simulink model "draft2"  (R2020b)
settings: Solver=VariableStepAuto  StartTime=0.0  StopTime=10.0  FixedStep=0.0001  MaxStep=0.2  RelTol=1e-3  AbsTol=1e-3  EnableMultiTasking=on
model workspace (MAT data in the model file):
  c = 0.1
  k : Simulink.Parameter (value not decoded)
libraries: nesl_utility x118, sm_lib x40, simulink x5, simulink_extras x5, fl_lib x1
(part 5 of 5)

== system draft2/T8/LB torque feedback L4 ==
  Gain4 : Gain  Gain=-1
  PS-Simulink Converter8 : nesl_utility/PS-Simulink Converter  PhysicalDomain=network_engine_domain  SubClassName=ps_output  LeftPortType=input  RightPortType=output  PseudoPeriodic=off  Frequencies=[]  Unit=inherit  AffineConversion=off
  Simulink-PS Converter5 : nesl_utility/Simulink-PS Converter  PhysicalDomain=network_engine_domain  SubClassName=ps_input  LeftPortType=input  RightPortType=output  PseudoPeriodic=off  Frequencies=[]  NoiseDistribution=none  NoiseParameters=[]  Unit=1  AffineConversion=off  FilteringAndDerivatives=provide  SimscapeFilterOrder=1  InputFilterTimeConstant=0.001  UdotUserProvided=0
  peacewise torque profile4 : MATLAB Function  TreatAsAtomicUnit=on
  LB rot : PMIOPort  Side=Left
  LB torque : PMIOPort  Port=2  Side=Right
  wires:
  peacewise torque profile4/1(torque) -> Gain4/1
  PS-Simulink Converter8/1 -> peacewise torque profile4/1(u)
  Gain4/1 -> Simulink-PS Converter5/1
  connections:
  LB rot/RConn1 -- PS-Simulink Converter8/LConn1
  Simulink-PS Converter5/RConn1 -- LB torque/RConn1

== system draft2/T9/AR torque feedback L4 ==
  Gain5 : Gain  Gain=-1
  PS-Simulink Converter9 : nesl_utility/PS-Simulink Converter  PhysicalDomain=network_engine_domain  SubClassName=ps_output  LeftPortType=input  RightPortType=output  PseudoPeriodic=off  Frequencies=[]  Unit=inherit  AffineConversion=off
  Simulink-PS Converter6 : nesl_utility/Simulink-PS Converter  PhysicalDomain=network_engine_domain  SubClassName=ps_input  LeftPortType=input  RightPortType=output  PseudoPeriodic=off  Frequencies=[]  NoiseDistribution=none  NoiseParameters=[]  Unit=1  AffineConversion=off  FilteringAndDerivatives=provide  SimscapeFilterOrder=1  InputFilterTimeConstant=0.001  UdotUserProvided=0
  peacewise torque profile5 : MATLAB Function  TreatAsAtomicUnit=on
  AR rot : PMIOPort  Side=Left
  AR torque : PMIOPort  Port=2  Side=Right
  wires:
  PS-Simulink Converter9/1 -> peacewise torque profile5/1(u)
  peacewise torque profile5/1(torque) -> Gain5/1
  Gain5/1 -> Simulink-PS Converter6/1
  connections:
  PS-Simulink Converter9/LConn1 -- AR rot/RConn1
  AR torque/RConn1 -- Simulink-PS Converter6/RConn1

== system draft2/T9/FE torque feedback L4 ==
  Gain7 : Gain  Gain=-1
  PS-Simulink Converter5 : nesl_utility/PS-Simulink Converter  PhysicalDomain=network_engine_domain  SubClassName=ps_output  LeftPortType=input  RightPortType=output  PseudoPeriodic=off  Frequencies=[]  Unit=inherit  AffineConversion=off
  Simulink-PS Converter4 : nesl_utility/Simulink-PS Converter  PhysicalDomain=network_engine_domain  SubClassName=ps_input  LeftPortType=input  RightPortType=output  PseudoPeriodic=off  Frequencies=[]  NoiseDistribution=none  NoiseParameters=[]  Unit=1  AffineConversion=off  FilteringAndDerivatives=provide  SimscapeFilterOrder=1  InputFilterTimeConstant=0.001  UdotUserProvided=0
  peacewise torque profile1 : MATLAB Function  TreatAsAtomicUnit=on
  FE rot : PMIOPort  Side=Left
  FE torque : PMIOPort  Port=2  Side=Right
  wires:
  PS-Simulink Converter5/1 -> peacewise torque profile1/1(u)
  peacewise torque profile1/1(torque) -> Gain7/1
  Gain7/1 -> Simulink-PS Converter4/1
  connections:
  FE rot/RConn1 -- PS-Simulink Converter5/LConn1
  FE torque/RConn1 -- Simulink-PS Converter4/RConn1

== system draft2/T9/LB torque feedback L4 ==
  Gain4 : Gain  Gain=-1
  PS-Simulink Converter8 : nesl_utility/PS-Simulink Converter  PhysicalDomain=network_engine_domain  SubClassName=ps_output  LeftPortType=input  RightPortType=output  PseudoPeriodic=off  Frequencies=[]  Unit=inherit  AffineConversion=off
  Simulink-PS Converter5 : nesl_utility/Simulink-PS Converter  PhysicalDomain=network_engine_domain  SubClassName=ps_input  LeftPortType=input  RightPortType=output  PseudoPeriodic=off  Frequencies=[]  NoiseDistribution=none  NoiseParameters=[]  Unit=1  AffineConversion=off  FilteringAndDerivatives=provide  SimscapeFilterOrder=1  InputFilterTimeConstant=0.001  UdotUserProvided=0
  peacewise torque profile4 : MATLAB Function  TreatAsAtomicUnit=on
  LB rot : PMIOPort  Side=Left
  LB torque : PMIOPort  Port=2  Side=Right
  wires:
  Gain4/1 -> Simulink-PS Converter5/1
  PS-Simulink Converter8/1 -> peacewise torque profile4/1(u)
  peacewise torque profile4/1(torque) -> Gain4/1
  connections:
  Simulink-PS Converter5/RConn1 -- LB torque/RConn1
  LB rot/RConn1 -- PS-Simulink Converter8/LConn1

== matlab function draft2/L1/LB torque feedback L4/peacewise torque profile4 ==
  data: u input; torque output
function torque = T(u)
torque = 0;
if (u >= 15)
    torque= -0.0015*1*(57.295*15)^4 + 0.1326*(57.295*15)^3 -0.3477*(57.295*15)^2 + 0.499*(57.295*15);
 
elseif (u >= -15 && u<= 15)
    torque= -0.0015*(57.295*u)^4 + 0.1326*(57.295*u)^3 -0.3477*(57.295*u)^2 + 0.499*(57.295*u)   ;
    
elseif (u <= -15)
   torque= -0.0015*1*(57.295*-15)^4 + 0.1326*(57.295*-15)^3 -0.3477*(57.295*-15)^2 + 0.499*(57.295*-15);
end

== matlab function draft2/T12/AR torque feedback L4/peacewise torque profile5 ==
  data: u input; torque output
function torque = T(u)
torque = 0;
if (u >= 15)
    torque= -0.0015*1*(57.295*15)^4 + 0.1326*(57.295*15)^3 -0.3477*(57.295*15)^2 + 0.499*(57.295*15);
 
elseif (u >= -15 && u<= 15)
    torque= -0.0015*(57.295*u)^4 + 0.1326*(57.295*u)^3 -0.3477*(57.295*u)^2 + 0.499*(57.295*u)   ;
    
elseif (u <= -15)
   torque= -0.0015*1*(57.295*-15)^4 + 0.1326*(57.295*-15)^3 -0.3477*(57.295*-15)^2 + 0.499*(57.295*-15);
end

== matlab function draft2/T12/FE torque feedback L4/peacewise torque profile1 ==
  data: u input; torque output
function torque = T(u)
torque = 0;
if (u >= 15)
    torque= -0.0015*1*(57.295*15)^4 + 0.1326*(57.295*15)^3 -0.3477*(57.295*15)^2 + 0.499*(57.295*15);
 
elseif (u >= -15 && u<= 15)
    torque= -0.0015*(57.295*u)^4 + 0.1326*(57.295*u)^3 -0.3477*(57.295*u)^2 + 0.499*(57.295*u)   ;
    
elseif (u <= -15)
   torque= -0.0015*1*(57.295*-15)^4 + 0.1326*(57.295*-15)^3 -0.3477*(57.295*-15)^2 + 0.499*(57.295*-15);
end

== matlab function draft2/T12/LB torque feedback L4/peacewise torque profile4 ==
  data: u input; torque output
function torque = T(u)
torque = 0;
if (u >= 15)
    torque= -0.0015*1*(57.295*15)^4 + 0.1326*(57.295*15)^3 -0.3477*(57.295*15)^2 + 0.499*(57.295*15);
 
elseif (u >= -15 && u<= 15)
    torque= -0.0015*(57.295*u)^4 + 0.1326*(57.295*u)^3 -0.3477*(57.295*u)^2 + 0.499*(57.295*u)   ;
    
elseif (u <= -15)
   torque= -0.0015*1*(57.295*-15)^4 + 0.1326*(57.295*-15)^3 -0.3477*(57.295*-15)^2 + 0.499*(57.295*-15);
end

== matlab function draft2/T11/AR torque feedback L4/peacewise torque profile5 ==
  data: u input; torque output
function torque = T(u)
torque = 0;
if (u >= 15)
    torque= -0.0015*1*(57.295*15)^4 + 0.1326*(57.295*15)^3 -0.3477*(57.295*15)^2 + 0.499*(57.295*15);
 
elseif (u >= -15 && u<= 15)
    torque= -0.0015*(57.295*u)^4 + 0.1326*(57.295*u)^3 -0.3477*(57.295*u)^2 + 0.499*(57.295*u)   ;
    
elseif (u <= -15)
   torque= -0.0015*1*(57.295*-15)^4 + 0.1326*(57.295*-15)^3 -0.3477*(57.295*-15)^2 + 0.499*(57.295*-15);
end

== matlab function draft2/L5/FE torque feedback L5/peacewise torque profile (+- 15 deg) ==
  data: u input; torque output
function torque = T(u)
torque = 0;
if (u >= 15)
    torque= -0.0015*1*(57.295*15)^4 + 0.1326*(57.295*15)^3 -0.3477*(57.295*15)^2 + 0.499*(57.295*15);
 
elseif (u >= -15 && u<= 15)
    torque= -0.0015*(57.295*u)^4 + 0.1326*(57.295*u)^3 -0.3477*(57.295*u)^2 + 0.499*(57.295*u)   ;
    
elseif (u <= -15)
   torque= -0.0015*1*(57.295*-15)^4 + 0.1326*(57.295*-15)^3 -0.3477*(57.295*-15)^2 + 0.499*(57.295*-15);
end

== matlab function draft2/T11/FE torque feedback L4/peacewise torque profile1 ==
  data: u input; torque output
function torque = T(u)
torque = 0;
if (u >= 15)
    torque= -0.0015*1*(57.295*15)^4 + 0.1326*(57.295*15)^3 -0.3477*(57.295*15)^2 + 0.499*(57.295*15);
 
elseif (u >= -15 && u<= 15)
    torque= -0.0015*(57.295*u)^4 + 0.1326*(57.295*u)^3 -0.3477*(57.295*u)^2 + 0.499*(57.295*u)   ;
    
elseif (u <= -15)
   torque= -0.0015*1*(57.295*-15)^4 + 0.1326*(57.295*-15)^3 -0.3477*(57.295*-15)^2 + 0.499*(57.295*-15);
end

== matlab function draft2/T11/LB torque feedback L4/peacewise torque profile4 ==
  data: u input; torque output
function torque = T(u)
torque = 0;
if (u >= 15)
    torque= -0.0015*1*(57.295*15)^4 + 0.1326*(57.295*15)^3 -0.3477*(57.295*15)^2 + 0.499*(57.295*15);
 
elseif (u >= -15 && u<= 15)
    torque= -0.0015*(57.295*u)^4 + 0.1326*(57.295*u)^3 -0.3477*(57.295*u)^2 + 0.499*(57.295*u)   ;
    
elseif (u <= -15)
   torque= -0.0015*1*(57.295*-15)^4 + 0.1326*(57.295*-15)^3 -0.3477*(57.295*-15)^2 + 0.499*(57.295*-15);
end

== matlab function draft2/T10/AR torque feedback L4/peacewise torque profile5 ==
  data: u input; torque output
function torque = T(u)
torque = 0;
if (u >= 15)
    torque= -0.0015*1*(57.295*15)^4 + 0.1326*(57.295*15)^3 -0.3477*(57.295*15)^2 + 0.499*(57.295*15);
 
elseif (u >= -15 && u<= 15)
    torque= -0.0015*(57.295*u)^4 + 0.1326*(57.295*u)^3 -0.3477*(57.295*u)^2 + 0.499*(57.295*u)   ;
    
elseif (u <= -15)
   torque= -0.0015*1*(57.295*-15)^4 + 0.1326*(57.295*-15)^3 -0.3477*(57.295*-15)^2 + 0.499*(57.295*-15);
end

== matlab function draft2/T10/FE torque feedback L4/peacewise torque profile1 ==
  data: u input; torque output
function torque = T(u)
torque = 0;
if (u >= 15)
    torque= -0.0015*1*(57.295*15)^4 + 0.1326*(57.295*15)^3 -0.3477*(57.295*15)^2 + 0.499*(57.295*15);
 
elseif (u >= -15 && u<= 15)
    torque= -0.0015*(57.295*u)^4 + 0.1326*(57.295*u)^3 -0.3477*(57.295*u)^2 + 0.499*(57.295*u)   ;
    
elseif (u <= -15)
   torque= -0.0015*1*(57.295*-15)^4 + 0.1326*(57.295*-15)^3 -0.3477*(57.295*-15)^2 + 0.499*(57.295*-15);
end

== matlab function draft2/T10/LB torque feedback L4/peacewise torque profile4 ==
  data: u input; torque output
function torque = T(u)
torque = 0;
if (u >= 15)
    torque= -0.0015*1*(57.295*15)^4 + 0.1326*(57.295*15)^3 -0.3477*(57.295*15)^2 + 0.499*(57.295*15);
 
elseif (u >= -15 && u<= 15)
    torque= -0.0015*(57.295*u)^4 + 0.1326*(57.295*u)^3 -0.3477*(57.295*u)^2 + 0.499*(57.295*u)   ;
    
elseif (u <= -15)
   torque= -0.0015*1*(57.295*-15)^4 + 0.1326*(57.295*-15)^3 -0.3477*(57.295*-15)^2 + 0.499*(57.295*-15);
end

== matlab function draft2/T9/AR torque feedback L4/peacewise torque profile5 ==
  data: u input; torque output
function torque = T(u)
torque = 0;
if (u >= 15)
    torque= -0.0015*1*(57.295*15)^4 + 0.1326*(57.295*15)^3 -0.3477*(57.295*15)^2 + 0.499*(57.295*15);
 
elseif (u >= -15 && u<= 15)
    torque= -0.0015*(57.295*u)^4 + 0.1326*(57.295*u)^3 -0.3477*(57.295*u)^2 + 0.499*(57.295*u)   ;
    
elseif (u <= -15)
   torque= -0.0015*1*(57.295*-15)^4 + 0.1326*(57.295*-15)^3 -0.3477*(57.295*-15)^2 + 0.499*(57.295*-15);
end

== matlab function draft2/T9/FE torque feedback L4/peacewise torque profile1 ==
  data: u input; torque output
function torque = T(u)
torque = 0;
if (u >= 15)
    torque= -0.0015*1*(57.295*15)^4 + 0.1326*(57.295*15)^3 -0.3477*(57.295*15)^2 + 0.499*(57.295*15);
 
elseif (u >= -15 && u<= 15)
    torque= -0.0015*(57.295*u)^4 + 0.1326*(57.295*u)^3 -0.3477*(57.295*u)^2 + 0.499*(57.295*u)   ;
    
elseif (u <= -15)
   torque= -0.0015*1*(57.295*-15)^4 + 0.1326*(57.295*-15)^3 -0.3477*(57.295*-15)^2 + 0.499*(57.295*-15);
end

== matlab function draft2/T9/LB torque feedback L4/peacewise torque profile4 ==
  data: u input; torque output
function torque = T(u)
torque = 0;
if (u >= 15)
    torque= -0.0015*1*(57.295*15)^4 + 0.1326*(57.295*15)^3 -0.3477*(57.295*15)^2 + 0.499*(57.295*15);
 
elseif (u >= -15 && u<= 15)
    torque= -0.0015*(57.295*u)^4 + 0.1326*(57.295*u)^3 -0.3477*(57.295*u)^2 + 0.499*(57.295*u)   ;
    
elseif (u <= -15)
   torque= -0.0015*1*(57.295*-15)^4 + 0.1326*(57.295*-15)^3 -0.3477*(57.295*-15)^2 + 0.499*(57.295*-15);
end

== matlab function draft2/T8/AR torque feedback L4/peacewise torque profile5 ==
  data: u input; torque output
function torque = T(u)
torque = 0;
if (u >= 15)
    torque= -0.0015*1*(57.295*15)^4 + 0.1326*(57.295*15)^3 -0.3477*(57.295*15)^2 + 0.499*(57.295*15);
 
elseif (u >= -15 && u<= 15)
    torque= -0.0015*(57.295*u)^4 + 0.1326*(57.295*u)^3 -0.3477*(57.295*u)^2 + 0.499*(57.295*u)   ;
    
elseif (u <= -15)
   torque= -0.0015*1*(57.295*-15)^4 + 0.1326*(57.295*-15)^3 -0.3477*(57.295*-15)^2 + 0.499*(57.295*-15);
end

== matlab function draft2/T8/FE torque feedback L4/peacewise torque profile1 ==
  data: u input; torque output
function torque = T(u)
torque = 0;
if (u >= 15)
    torque= -0.0015*1*(57.295*15)^4 + 0.1326*(57.295*15)^3 -0.3477*(57.295*15)^2 + 0.499*(57.295*15);
 
elseif (u >= -15 && u<= 15)
    torque= -0.0015*(57.295*u)^4 + 0.1326*(57.295*u)^3 -0.3477*(57.295*u)^2 + 0.499*(57.295*u)   ;
    
elseif (u <= -15)
   torque= -0.0015*1*(57.295*-15)^4 + 0.1326*(57.295*-15)^3 -0.3477*(57.295*-15)^2 + 0.499*(57.295*-15);
end

== matlab function draft2/L5/LB torque feedback L5/peacewise torque profile2 ==
  data: u input; torque output
function torque = T(u)
torque = 0;
if (u >= 15)
    torque= -0.0015*1*(57.295*15)^4 + 0.1326*(57.295*15)^3 -0.3477*(57.295*15)^2 + 0.499*(57.295*15);
 
elseif (u >= -15 && u<= 15)
    torque= -0.0015*(57.295*u)^4 + 0.1326*(57.295*u)^3 -0.3477*(57.295*u)^2 + 0.499*(57.295*u)   ;
    
elseif (u <= -15)
   torque= -0.0015*1*(57.295*-15)^4 + 0.1326*(57.295*-15)^3 -0.3477*(57.295*-15)^2 + 0.499*(57.295*-15);
end

== matlab function draft2/T8/LB torque feedback L4/peacewise torque profile4 ==
  data: u input; torque output
function torque = T(u)
torque = 0;
if (u >= 15)
    torque= -0.0015*1*(57.295*15)^4 + 0.1326*(57.295*15)^3 -0.3477*(57.295*15)^2 + 0.499*(57.295*15);
 
elseif (u >= -15 && u<= 15)
    torque= -0.0015*(57.295*u)^4 + 0.1326*(57.295*u)^3 -0.3477*(57.295*u)^2 + 0.499*(57.295*u)   ;
    
elseif (u <= -15)
   torque= -0.0015*1*(57.295*-15)^4 + 0.1326*(57.295*-15)^3 -0.3477*(57.295*-15)^2 + 0.499*(57.295*-15);
end

== matlab function draft2/T7/AR torque feedback L4/peacewise torque profile5 ==
  data: u input; torque output
function torque = T(u)
torque = 0;
if (u >= 15)
    torque= -0.0015*1*(57.295*15)^4 + 0.1326*(57.295*15)^3 -0.3477*(57.295*15)^2 + 0.499*(57.295*15);
 
elseif (u >= -15 && u<= 15)
    torque= -0.0015*(57.295*u)^4 + 0.1326*(57.295*u)^3 -0.3477*(57.295*u)^2 + 0.499*(57.295*u)   ;
    
elseif (u <= -15)
   torque= -0.0015*1*(57.295*-15)^4 + 0.1326*(57.295*-15)^3 -0.3477*(57.295*-15)^2 + 0.499*(57.295*-15);
end

== matlab function draft2/T7/FE torque feedback L4/peacewise torque profile1 ==
  data: u input; torque output
function torque = T(u)
torque = 0;
if (u >= 15)
    torque= -0.0015*1*(57.295*15)^4 + 0.1326*(57.295*15)^3 -0.3477*(57.295*15)^2 + 0.499*(57.295*15);
 
elseif (u >= -15 && u<= 15)
    torque= -0.0015*(57.295*u)^4 + 0.1326*(57.295*u)^3 -0.3477*(57.295*u)^2 + 0.499*(57.295*u)   ;
    
elseif (u <= -15)
   torque= -0.0015*1*(57.295*-15)^4 + 0.1326*(57.295*-15)^3 -0.3477*(57.295*-15)^2 + 0.499*(57.295*-15);
end

== matlab function draft2/T7/LB torque feedback L4/peacewise torque profile4 ==
  data: u input; torque output
function torque = T(u)
torque = 0;
if (u >= 15)
    torque= -0.0015*1*(57.295*15)^4 + 0.1326*(57.295*15)^3 -0.3477*(57.295*15)^2 + 0.499*(57.295*15);
 
elseif (u >= -15 && u<= 15)
    torque= -0.0015*(57.295*u)^4 + 0.1326*(57.295*u)^3 -0.3477*(57.295*u)^2 + 0.499*(57.295*u)   ;
    
elseif (u <= -15)
   torque= -0.0015*1*(57.295*-15)^4 + 0.1326*(57.295*-15)^3 -0.3477*(57.295*-15)^2 + 0.499*(57.295*-15);
end

== matlab function draft2/T6/AR torque feedback L4/peacewise torque profile5 ==
  data: u input; torque output
function torque = T(u)
torque = 0;
if (u >= 15)
    torque= -0.0015*1*(57.295*15)^4 + 0.1326*(57.295*15)^3 -0.3477*(57.295*15)^2 + 0.499*(57.295*15);
 
elseif (u >= -15 && u<= 15)
    torque= -0.0015*(57.295*u)^4 + 0.1326*(57.295*u)^3 -0.3477*(57.295*u)^2 + 0.499*(57.295*u)   ;
    
elseif (u <= -15)
   torque= -0.0015*1*(57.295*-15)^4 + 0.1326*(57.295*-15)^3 -0.3477*(57.295*-15)^2 + 0.499*(57.295*-15);
end

== matlab function draft2/T6/FE torque feedback L4/peacewise torque profile1 ==
  data: u input; torque output
function torque = T(u)
torque = 0;
if (u >= 15)
    torque= -0.0015*1*(57.295*15)^4 + 0.1326*(57.295*15)^3 -0.3477*(57.295*15)^2 + 0.499*(57.295*15);
 
elseif (u >= -15 && u<= 15)
    torque= -0.0015*(57.295*u)^4 + 0.1326*(57.295*u)^3 -0.3477*(57.295*u)^2 + 0.499*(57.295*u)   ;
    
elseif (u <= -15)
   torque= -0.0015*1*(57.295*-15)^4 + 0.1326*(57.295*-15)^3 -0.3477*(57.295*-15)^2 + 0.499*(57.295*-15);
end

== matlab function draft2/T6/LB torque feedback L4/peacewise torque profile4 ==
  data: u input; torque output
function torque = T(u)
torque = 0;
if (u >= 15)
    torque= -0.0015*1*(57.295*15)^4 + 0.1326*(57.295*15)^3 -0.3477*(57.295*15)^2 + 0.499*(57.295*15);
 
elseif (u >= -15 && u<= 15)
    torque= -0.0015*(57.295*u)^4 + 0.1326*(57.295*u)^3 -0.3477*(57.295*u)^2 + 0.499*(57.295*u)   ;
    
elseif (u <= -15)
   torque= -0.0015*1*(57.295*-15)^4 + 0.1326*(57.295*-15)^3 -0.3477*(57.295*-15)^2 + 0.499*(57.295*-15);
end

== matlab function draft2/T5/AR torque feedback L4/peacewise torque profile5 ==
  data: u input; torque output
function torque = T(u)
torque = 0;
if (u >= 15)
    torque= -0.0015*1*(57.295*15)^4 + 0.1326*(57.295*15)^3 -0.3477*(57.295*15)^2 + 0.499*(57.295*15);
 
elseif (u >= -15 && u<= 15)
    torque= -0.0015*(57.295*u)^4 + 0.1326*(57.295*u)^3 -0.3477*(57.295*u)^2 + 0.499*(57.295*u)   ;
    
elseif (u <= -15)
   torque= -0.0015*1*(57.295*-15)^4 + 0.1326*(57.295*-15)^3 -0.3477*(57.295*-15)^2 + 0.499*(57.295*-15);
end

== matlab function draft2/T5/FE torque feedback L4/peacewise torque profile1 ==
  data: u input; torque output
function torque = T(u)
torque = 0;
if (u >= 15)
    torque= -0.0015*1*(57.295*15)^4 + 0.1326*(57.295*15)^3 -0.3477*(57.295*15)^2 + 0.499*(57.295*15);
 
elseif (u >= -15 && u<= 15)
    torque= -0.0015*(57.295*u)^4 + 0.1326*(57.295*u)^3 -0.3477*(57.295*u)^2 + 0.499*(57.295*u)   ;
    
elseif (u <= -15)
   torque= -0.0015*1*(57.295*-15)^4 + 0.1326*(57.295*-15)^3 -0.3477*(57.295*-15)^2 + 0.499*(57.295*-15);
end

== matlab function draft2/T5/LB torque feedback L4/peacewise torque profile4 ==
  data: u input; torque output
function torque = T(u)
torque = 0;
if (u >= 15)
    torque= -0.0015*1*(57.295*15)^4 + 0.1326*(57.295*15)^3 -0.3477*(57.295*15)^2 + 0.499*(57.295*15);
 
elseif (u >= -15 && u<= 15)
    torque= -0.0015*(57.295*u)^4 + 0.1326*(57.295*u)^3 -0.3477*(57.295*u)^2 + 0.499*(57.295*u)   ;
    
elseif (u <= -15)
   torque= -0.0015*1*(57.295*-15)^4 + 0.1326*(57.295*-15)^3 -0.3477*(57.295*-15)^2 + 0.499*(57.295*-15);
end

== matlab function draft2/L5/AR torque feedback L5/peacewise torque profile3 ==
  data: u input; torque output
function torque = T(u)
torque = 0;
if (u >= 15)
    torque= -0.0015*1*(57.295*15)^4 + 0.1326*(57.295*15)^3 -0.3477*(57.295*15)^2 + 0.499*(57.295*15);
 
elseif (u >= -15 && u<= 15)
    torque= -0.0015*(57.295*u)^4 + 0.1326*(57.295*u)^3 -0.3477*(57.295*u)^2 + 0.499*(57.295*u)   ;
    
elseif (u <= -15)
   torque= -0.0015*1*(57.295*-15)^4 + 0.1326*(57.295*-15)^3 -0.3477*(57.295*-15)^2 + 0.499*(57.295*-15);
end

== matlab function draft2/T4/AR torque feedback L4/peacewise torque profile5 ==
  data: u input; torque output
function torque = T(u)
torque = 0;
if (u >= 15)
    torque= -0.0015*1*(57.295*15)^4 + 0.1326*(57.295*15)^3 -0.3477*(57.295*15)^2 + 0.499*(57.295*15);
 
elseif (u >= -15 && u<= 15)
    torque= -0.0015*(57.295*u)^4 + 0.1326*(57.295*u)^3 -0.3477*(57.295*u)^2 + 0.499*(57.295*u)   ;
    
elseif (u <= -15)
   torque= -0.0015*1*(57.295*-15)^4 + 0.1326*(57.295*-15)^3 -0.3477*(57.295*-15)^2 + 0.499*(57.295*-15);
end

== matlab function draft2/T4/FE torque feedback L4/peacewise torque profile1 ==
  data: u input; torque output
function torque = T(u)
torque = 0;
if (u >= 15)
    torque= -0.0015*1*(57.295*15)^4 + 0.1326*(57.295*15)^3 -0.3477*(57.295*15)^2 + 0.499*(57.295*15);
 
elseif (u >= -15 && u<= 15)
    torque= -0.0015*(57.295*u)^4 + 0.1326*(57.295*u)^3 -0.3477*(57.295*u)^2 + 0.499*(57.295*u)   ;
    
elseif (u <= -15)
   torque= -0.0015*1*(57.295*-15)^4 + 0.1326*(57.295*-15)^3 -0.3477*(57.295*-15)^2 + 0.499*(57.295*-15);
end

== matlab function draft2/T4/LB torque feedback L4/peacewise torque profile4 ==
  data: u input; torque output
function torque = T(u)
torque = 0;
if (u >= 15)
    torque= -0.0015*1*(57.295*15)^4 + 0.1326*(57.295*15)^3 -0.3477*(57.295*15)^2 + 0.499*(57.295*15);
 
elseif (u >= -15 && u<= 15)
    torque= -0.0015*(57.295*u)^4 + 0.1326*(57.295*u)^3 -0.3477*(57.295*u)^2 + 0.499*(57.295*u)   ;
    
elseif (u <= -15)
   torque= -0.0015*1*(57.295*-15)^4 + 0.1326*(57.295*-15)^3 -0.3477*(57.295*-15)^2 + 0.499*(57.295*-15);
end

== matlab function draft2/T3/AR torque feedback L4/peacewise torque profile5 ==
  data: u input; torque output
function torque = T(u)
torque = 0;
if (u >= 15)
    torque= -0.0015*1*(57.295*15)^4 + 0.1326*(57.295*15)^3 -0.3477*(57.295*15)^2 + 0.499*(57.295*15);
 
elseif (u >= -15 && u<= 15)
    torque= -0.0015*(57.295*u)^4 + 0.1326*(57.295*u)^3 -0.3477*(57.295*u)^2 + 0.499*(57.295*u)   ;
    
elseif (u <= -15)
   torque= -0.0015*1*(57.295*-15)^4 + 0.1326*(57.295*-15)^3 -0.3477*(57.295*-15)^2 + 0.499*(57.295*-15);
end

== matlab function draft2/T3/FE torque feedback L4/peacewise torque profile1 ==
  data: u input; torque output
function torque = T(u)
torque = 0;
if (u >= 15)
    torque= -0.0015*1*(57.295*15)^4 + 0.1326*(57.295*15)^3 -0.3477*(57.295*15)^2 + 0.499*(57.295*15);
 
elseif (u >= -15 && u<= 15)
    torque= -0.0015*(57.295*u)^4 + 0.1326*(57.295*u)^3 -0.3477*(57.295*u)^2 + 0.499*(57.295*u)   ;
    
elseif (u <= -15)
   torque= -0.0015*1*(57.295*-15)^4 + 0.1326*(57.295*-15)^3 -0.3477*(57.295*-15)^2 + 0.499*(57.295*-15);
end

== matlab function draft2/T3/LB torque feedback L4/peacewise torque profile4 ==
  data: u input; torque output
function torque = T(u)
torque = 0;
if (u >= 15)
    torque= -0.0015*1*(57.295*15)^4 + 0.1326*(57.295*15)^3 -0.3477*(57.295*15)^2 + 0.499*(57.295*15);
 
elseif (u >= -15 && u<= 15)
    torque= -0.0015*(57.295*u)^4 + 0.1326*(57.295*u)^3 -0.3477*(57.295*u)^2 + 0.499*(57.295*u)   ;
    
elseif (u <= -15)
   torque= -0.0015*1*(57.295*-15)^4 + 0.1326*(57.295*-15)^3 -0.3477*(57.295*-15)^2 + 0.499*(57.295*-15);
end

== matlab function draft2/T2/AR torque feedback L4/peacewise torque profile5 ==
  data: u input; torque output
function torque = T(u)
torque = 0;
if (u >= 15)
    torque= -0.0015*1*(57.295*15)^4 + 0.1326*(57.295*15)^3 -0.3477*(57.295*15)^2 + 0.499*(57.295*15);
 
elseif (u >= -15 && u<= 15)
    torque= -0.0015*(57.295*u)^4 + 0.1326*(57.295*u)^3 -0.3477*(57.295*u)^2 + 0.499*(57.295*u)   ;
    
elseif (u <= -15)
   torque= -0.0015*1*(57.295*-15)^4 + 0.1326*(57.295*-15)^3 -0.3477*(57.295*-15)^2 + 0.499*(57.295*-15);
end

== matlab function draft2/T2/FE torque feedback L4/peacewise torque profile1 ==
  data: u input; torque output
function torque = T(u)
torque = 0;
if (u >= 15)
    torque= -0.0015*1*(57.295*15)^4 + 0.1326*(57.295*15)^3 -0.3477*(57.295*15)^2 + 0.499*(57.295*15);
 
elseif (u >= -15 && u<= 15)
    torque= -0.0015*(57.295*u)^4 + 0.1326*(57.295*u)^3 -0.3477*(57.295*u)^2 + 0.499*(57.295*u)   ;
    
elseif (u <= -15)
   torque= -0.0015*1*(57.295*-15)^4 + 0.1326*(57.295*-15)^3 -0.3477*(57.295*-15)^2 + 0.499*(57.295*-15);
end

== matlab function draft2/T2/LB torque feedback L4/peacewise torque profile4 ==
  data: u input; torque output
function torque = T(u)
torque = 0;
if (u >= 15)
    torque= -0.0015*1*(57.295*15)^4 + 0.1326*(57.295*15)^3 -0.3477*(57.295*15)^2 + 0.499*(57.295*15);
 
elseif (u >= -15 && u<= 15)
    torque= -0.0015*(57.295*u)^4 + 0.1326*(57.295*u)^3 -0.3477*(57.295*u)^2 + 0.499*(57.295*u)   ;
    
elseif (u <= -15)
   torque= -0.0015*1*(57.295*-15)^4 + 0.1326*(57.295*-15)^3 -0.3477*(57.295*-15)^2 + 0.499*(57.295*-15);
end

== matlab function draft2/T1/AR torque feedback L4/peacewise torque profile5 ==
  data: u input; torque output
function torque = T(u)
torque = 0;
if (u >= 15)
    torque= -0.0015*1*(57.295*15)^4 + 0.1326*(57.295*15)^3 -0.3477*(57.295*15)^2 + 0.499*(57.295*15);
 
elseif (u >= -15 && u<= 15)
    torque= -0.0015*(57.295*u)^4 + 0.1326*(57.295*u)^3 -0.3477*(57.295*u)^2 + 0.499*(57.295*u)   ;
    
elseif (u <= -15)
   torque= -0.0015*1*(57.295*-15)^4 + 0.1326*(57.295*-15)^3 -0.3477*(57.295*-15)^2 + 0.499*(57.295*-15);
end

== matlab function draft2/L4/LB torque feedback L4/peacewise torque profile4 ==
  data: u input; torque output
function torque = T(u)
torque = 0;
if (u >= 15)
    torque= -0.0015*1*(57.295*15)^4 + 0.1326*(57.295*15)^3 -0.3477*(57.295*15)^2 + 0.499*(57.295*15);
 
elseif (u >= -15 && u<= 15)
    torque= -0.0015*(57.295*u)^4 + 0.1326*(57.295*u)^3 -0.3477*(57.295*u)^2 + 0.499*(57.295*u)   ;
    
elseif (u <= -15)
   torque= -0.0015*1*(57.295*-15)^4 + 0.1326*(57.295*-15)^3 -0.3477*(57.295*-15)^2 + 0.499*(57.295*-15);
end

== matlab function draft2/T1/FE torque feedback L4/peacewise torque profile1 ==
  data: u input; torque output
function torque = T(u)
torque = 0;
if (u >= 15)
    torque= -0.0015*1*(57.295*15)^4 + 0.1326*(57.295*15)^3 -0.3477*(57.295*15)^2 + 0.499*(57.295*15);
 
elseif (u >= -15 && u<= 15)
    torque= -0.0015*(57.295*u)^4 + 0.1326*(57.295*u)^3 -0.3477*(57.295*u)^2 + 0.499*(57.295*u)   ;
    
elseif (u <= -15)
   torque= -0.0015*1*(57.295*-15)^4 + 0.1326*(57.295*-15)^3 -0.3477*(57.295*-15)^2 + 0.499*(57.295*-15);
end

== matlab function draft2/T1/LB torque feedback L4/peacewise torque profile4 ==
  data: u input; torque output
function torque = T(u)
torque = 0;
if (u >= 15)
    torque= -0.0015*1*(57.295*15)^4 + 0.1326*(57.295*15)^3 -0.3477*(57.295*15)^2 + 0.499*(57.295*15);
 
elseif (u >= -15 && u<= 15)
    torque= -0.0015*(57.295*u)^4 + 0.1326*(57.295*u)^3 -0.3477*(57.295*u)^2 + 0.499*(57.295*u)   ;
    
elseif (u <= -15)
   torque= -0.0015*1*(57.295*-15)^4 + 0.1326*(57.295*-15)^3 -0.3477*(57.295*-15)^2 + 0.499*(57.295*-15);
end

== matlab function draft2/L4/AR torque feedback L4/peacewise torque profile5 ==
  data: u input; torque output
function torque = T(u)
torque = 0;
if (u >= 15)
    torque= -0.0015*1*(57.295*15)^4 + 0.1326*(57.295*15)^3 -0.3477*(57.295*15)^2 + 0.499*(57.295*15);
 
elseif (u >= -15 && u<= 15)
    torque= -0.0015*(57.295*u)^4 + 0.1326*(57.295*u)^3 -0.3477*(57.295*u)^2 + 0.499*(57.295*u)   ;
    
elseif (u <= -15)
   torque= -0.0015*1*(57.295*-15)^4 + 0.1326*(57.295*-15)^3 -0.3477*(57.295*-15)^2 + 0.499*(57.295*-15);
end

== matlab function draft2/L3/AR torque feedback L4/peacewise torque profile5 ==
  data: u input; torque output
function torque = T(u)
torque = 0;
if (u >= 15)
    torque= -0.0015*1*(57.295*15)^4 + 0.1326*(57.295*15)^3 -0.3477*(57.295*15)^2 + 0.499*(57.295*15);
 
elseif (u >= -15 && u<= 15)
    torque= -0.0015*(57.295*u)^4 + 0.1326*(57.295*u)^3 -0.3477*(57.295*u)^2 + 0.499*(57.295*u)   ;
    
elseif (u <= -15)
   torque= -0.0015*1*(57.295*-15)^4 + 0.1326*(57.295*-15)^3 -0.3477*(57.295*-15)^2 + 0.499*(57.295*-15);
end

== matlab function draft2/L3/FE torque feedback L4/peacewise torque profile1 ==
  data: u input; torque output
function torque = T(u)
torque = 0;
if (u >= 15)
    torque= -0.0015*1*(57.295*15)^4 + 0.1326*(57.295*15)^3 -0.3477*(57.295*15)^2 + 0.499*(57.295*15);
 
elseif (u >= -15 && u<= 15)
    torque= -0.0015*(57.295*u)^4 + 0.1326*(57.295*u)^3 -0.3477*(57.295*u)^2 + 0.499*(57.295*u)   ;
    
elseif (u <= -15)
   torque= -0.0015*1*(57.295*-15)^4 + 0.1326*(57.295*-15)^3 -0.3477*(57.295*-15)^2 + 0.499*(57.295*-15);
end

== matlab function draft2/L3/LB torque feedback L4/peacewise torque profile4 ==
  data: u input; torque output
function torque = T(u)
torque = 0;
if (u >= 15)
    torque= -0.0015*1*(57.295*15)^4 + 0.1326*(57.295*15)^3 -0.3477*(57.295*15)^2 + 0.499*(57.295*15);
 
elseif (u >= -15 && u<= 15)
    torque= -0.0015*(57.295*u)^4 + 0.1326*(57.295*u)^3 -0.3477*(57.295*u)^2 + 0.499*(57.295*u)   ;
    
elseif (u <= -15)
   torque= -0.0015*1*(57.295*-15)^4 + 0.1326*(57.295*-15)^3 -0.3477*(57.295*-15)^2 + 0.499*(57.295*-15);
end

== matlab function draft2/L4/FE torque feedback L4/peacewise torque profile1 ==
  data: u input; torque output
function torque = T(u)
torque = 0;
if (u >= 15)
    torque= -0.0015*1*(57.295*15)^4 + 0.1326*(57.295*15)^3 -0.3477*(57.295*15)^2 + 0.499*(57.295*15);
 
elseif (u >= -15 && u<= 15)
    torque= -0.0015*(57.295*u)^4 + 0.1326*(57.295*u)^3 -0.3477*(57.295*u)^2 + 0.499*(57.295*u)   ;
    
elseif (u <= -15)
   torque= -0.0015*1*(57.295*-15)^4 + 0.1326*(57.295*-15)^3 -0.3477*(57.295*-15)^2 + 0.499*(57.295*-15);
end

== matlab function draft2/L2/AR torque feedback L4/peacewise torque profile5 ==
  data: u input; torque output
function torque = T(u)
torque = 0;
if (u >= 15)
    torque= -0.0015*1*(57.295*15)^4 + 0.1326*(57.295*15)^3 -0.3477*(57.295*15)^2 + 0.499*(57.295*15);
 
elseif (u >= -15 && u<= 15)
    torque= -0.0015*(57.295*u)^4 + 0.1326*(57.295*u)^3 -0.3477*(57.295*u)^2 + 0.499*(57.295*u)   ;
    
elseif (u <= -15)
   torque= -0.0015*1*(57.295*-15)^4 + 0.1326*(57.295*-15)^3 -0.3477*(57.295*-15)^2 + 0.499*(57.295*-15);
end

== matlab function draft2/L2/FE torque feedback L4/peacewise torque profile1 ==
  data: u input; torque output
function torque = T(u)
torque = 0;
if (u >= 15)
    torque= -0.0015*1*(57.295*15)^4 + 0.1326*(57.295*15)^3 -0.3477*(57.295*15)^2 + 0.499*(57.295*15);
 
elseif (u >= -15 && u<= 15)
    torque= -0.0015*(57.295*u)^4 + 0.1326*(57.295*u)^3 -0.3477*(57.295*u)^2 + 0.499*(57.295*u)   ;
    
elseif (u <= -15)
   torque= -0.0015*1*(57.295*-15)^4 + 0.1326*(57.295*-15)^3 -0.3477*(57.295*-15)^2 + 0.499*(57.295*-15);
end

== matlab function draft2/L2/LB torque feedback L4/peacewise torque profile4 ==
  data: u input; torque output
function torque = T(u)
torque = 0;
if (u >= 15)
    torque= -0.0015*1*(57.295*15)^4 + 0.1326*(57.295*15)^3 -0.3477*(57.295*15)^2 + 0.499*(57.295*15);
 
elseif (u >= -15 && u<= 15)
    torque= -0.0015*(57.295*u)^4 + 0.1326*(57.295*u)^3 -0.3477*(57.295*u)^2 + 0.499*(57.295*u)   ;
    
elseif (u <= -15)
   torque= -0.0015*1*(57.295*-15)^4 + 0.1326*(57.295*-15)^3 -0.3477*(57.295*-15)^2 + 0.499*(57.295*-15);
end

== matlab function draft2/L1/AR torque feedback L4/peacewise torque profile5 ==
  data: u input; torque output
function torque = T(u)
torque = 0;
if (u >= 15)
    torque= -0.0015*1*(57.295*15)^4 + 0.1326*(57.295*15)^3 -0.3477*(57.295*15)^2 + 0.499*(57.295*15);
 
elseif (u >= -15 && u<= 15)
    torque= -0.0015*(57.295*u)^4 + 0.1326*(57.295*u)^3 -0.3477*(57.295*u)^2 + 0.499*(57.295*u)   ;
    
elseif (u <= -15)
   torque= -0.0015*1*(57.295*-15)^4 + 0.1326*(57.295*-15)^3 -0.3477*(57.295*-15)^2 + 0.499*(57.295*-15);
end

== matlab function draft2/L1/FE torque feedback L4/peacewise torque profile1 ==
  data: u input; torque output
function torque = T(u)
torque = 0;
if (u >= 15)
    torque= -0.0015*1*(57.295*15)^4 + 0.1326*(57.295*15)^3 -0.3477*(57.295*15)^2 + 0.499*(57.295*15);
 
elseif (u >= -15 && u<= 15)
    torque= -0.0015*(57.295*u)^4 + 0.1326*(57.295*u)^3 -0.3477*(57.295*u)^2 + 0.499*(57.295*u)   ;
    
elseif (u <= -15)
   torque= -0.0015*1*(57.295*-15)^4 + 0.1326*(57.295*-15)^3 -0.3477*(57.295*-15)^2 + 0.499*(57.295*-15);
end
